simulink model "ame532Project1_GimbalDynamicsModel"  (R2023a)
settings: Solver=ode4  StartTime=0.0  StopTime=10  FixedStep=0.01  RelTol=1e-3
model workspace (MAT data in the model file):
  theta : Simulink.Parameter (value not decoded)
values from neighbouring files (symbols this model uses):
  AR_s2 = b_s2/c_s2    [computeSurfacePos.m]
  AR_s3 = b_s3/c_s3    [computeSurfacePos.m]
  AR_s4 = b_s4/c_s4    [computeSurfacePos.m]
  AR_s5 = b_s5/c_s5    [computeSurfacePos.m]
  area_s2 = c_s2 * b_s2    [computeSurfacePos.m]
  area_s3 = c_s3 * b_s3    [computeSurfacePos.m]
  area_s4 = c_s4 * b_s4    [computeSurfacePos.m]
  area_s5 = c_s5 * b_s5    [computeSurfacePos.m]
  c_s2 = componentMassesAndGeom(3,2)    [computeSurfacePos.m]
  c_s3 = componentMassesAndGeom(4,2)    [computeSurfacePos.m]
  c_s4 = componentMassesAndGeom(1,2)    [computeSurfacePos.m]
  c_s5 = componentMassesAndGeom(2,2)    [computeSurfacePos.m]
undefined symbols (not defined in the file or in its folder): a0_s2, a0_s3, a0_s4, a0_s5, CD0_s2, CD0_s3, CD0_s4, CD0_s5, CDa_s2, CDa_s3, CDa_s4, CDa_s5, CL0_s2, CL0_s3, CL0_s4, CL0_s5, CM0_s2, CM0_s3, CM0_s4, CM0_s5, CMa_s2, CMa_s3, CMa_s4, CMa_s5, e_s2, e_s3, e_s4, e_s5, earthRadius, i_s2, i_s3, i_s4, i_s5, Jxx, Jxy, Jxz, Jyx, Jyy, Jyz, Jzx, Jzy, Jzz, LL, MM, n_s2, n_s3, n_s4, n_s5, NN, rEarth, ro, x_S2_B_B, x_S3_B_B, x_S4_B_B, x_S5_B_B
libraries: simulink_extras x34, matrix_library x22, aerolibutil x7, aerolibfltsims x4, vrlib x3, aerolibtransform2 x2, slpidlib x1, sharedutil x1, simulink x1
(part 3 of 4)

== system ame532Project1_GimbalDynamicsModel/JeoIMUmodel/Aero Forces and Moments/F&M Horiz Stab Surface (S3) ==
  v_B_E_B : Inport
  V_B_A_B (Relative AIr Speed) : Inport  Port=2
  Compute Aero Lift and Drag : MATLAB Function  TreatAsAtomicUnit=on
  Compute Aero Moment : MATLAB Function  TreatAsAtomicUnit=on
  Constant : Constant  Value=[AR_s3 i_s3 CL0_s3 CD0_s3 CDa_s3 a0_s3 e_s3 ro area_s3]
  Constant1 : Constant  Value=[CM0_s3; CMa_s3; c_s3]
  Constant2 : Constant  Value=n_s3
  Demux : Demux  Outputs=9
  Demux1 : Demux  Outputs=3
  F&M in Body : Subsystem
  momS3_B : Outport
  LiftAndDragForceS3_B : Outport  Port=2
  wires:
  Compute Aero Lift and Drag/2(liftSurf) -> F&M in Body/2(Lift)  "Lift Force w.r.t Wind"
  Compute Aero Moment/1(momSurf) -> F&M in Body/1(momSurf)  "Moment of Surface w.r.t Wind"
  Compute Aero Lift and Drag/3(dragSurf) -> F&M in Body/3(Drag)  "Drag Force w.r.t Wind"
  F&M in Body/2(LiftAndDragForceS3_B) -> LiftAndDragForceS3_B/1
  Compute Aero Lift and Drag/1(alphaLocal) -> Compute Aero Moment/2(alphaLocal)
  v_B_E_B/1 -> Compute Aero Lift and Drag/1(v_B_E_B), F&M in Body/4(v_B_E_B), Compute Aero Moment/1(v_B_E_B)
  F&M in Body/1(momS3_B) -> momS3_B/1
  V_B_A_B (Relative AIr Speed)/1 -> Compute Aero Lift and Drag/2(v_B_A_B)
  Constant/1 -> Demux/1
  Demux/1 -> Compute Aero Lift and Drag/3(AR_s3)  "AR_s3"
  Demux/2 -> Compute Aero Lift and Drag/4(i_s3)  "i_s3"
  Constant2/1 -> F&M in Body/5(n_s3), Compute Aero Lift and Drag/5(n_s3)  "n_s3"
  Demux/3 -> Compute Aero Lift and Drag/6(CL0_s3)  "CL0_s3"
  Demux/4 -> Compute Aero Lift and Drag/7(CD0_s3)  "CD0_s3"
  Demux/5 -> Compute Aero Lift and Drag/8(CDa_s3)  "CDa_s3"
  Demux/6 -> Compute Aero Lift and Drag/9(a0_s3)  "a0_s3"
  Demux/7 -> Compute Aero Lift and Drag/10(e_s3)  "e_s3"
  Demux/8 -> Compute Aero Moment/5(ro), Compute Aero Lift and Drag/11(ro)  "ro"
  Demux/9 -> Compute Aero Moment/6(area_s3), Compute Aero Lift and Drag/12(area_s3)  "area_s3"
  Constant1/1 -> Demux1/1
  Demux1/1 -> Compute Aero Moment/3(CM0_s3)  "CMo_s3"
  Demux1/2 -> Compute Aero Moment/4(CMa_s3)  "CMa_s3"
  Demux1/3 -> Compute Aero Moment/7(c_s3)  "c_s3"

== system ame532Project1_GimbalDynamicsModel/JeoIMUmodel/Aero Forces and Moments/F&M Right Wing and Servo Surface (S4) ==
  v_B_E_B : Inport
  V_B_A_B (Relative AIr Speed) : Inport  Port=2
  Compute Aero Lift and Drag : MATLAB Function  TreatAsAtomicUnit=on
  Compute Aero Moment : MATLAB Function  TreatAsAtomicUnit=on
  Constant : Constant  Value="[AR_s4 i_s4  CL0_s4 CD0_s4 CDa_s4 a0_s4 e_s4 ro area_s4]"
  Constant1 : Constant  Value=[CM0_s4; CMa_s4; c_s4]
  Demux : Demux  Outputs=9
  Demux1 : Demux  Outputs=3
  F&M in Body : Subsystem
  n_s4 : Constant  Value=n_s4
  momS4_B : Outport
  LiftAndDragForceS4_B : Outport  Port=2
  wires:
  Compute Aero Lift and Drag/2(liftSurf) -> F&M in Body/2(Lift)  "Lift Force w.r.t Wind"
  Compute Aero Moment/1(momSurf) -> F&M in Body/1(momSurf)  "Moment of Surface w.r.t Wind"
  Compute Aero Lift and Drag/3(dragSurf) -> F&M in Body/3(Drag)  "Drag Force w.r.t Wind"
  F&M in Body/2(LiftAndDragForceS4_B) -> LiftAndDragForceS4_B/1
  Compute Aero Lift and Drag/1(alphaLocal) -> Compute Aero Moment/2(alphaLocal)
  v_B_E_B/1 -> Compute Aero Lift and Drag/1(v_B_E_B), F&M in Body/4(v_B_E_B), Compute Aero Moment/1(v_B_E_B)
  F&M in Body/1(momS4_B) -> momS4_B/1
  V_B_A_B (Relative AIr Speed)/1 -> Compute Aero Lift and Drag/2(v_B_A_B)
  Constant/1 -> Demux/1
  Demux/1 -> Compute Aero Lift and Drag/3(AR_s4)  "AR_s4"
  Demux/2 -> Compute Aero Lift and Drag/4(i_s4)  "i_s4"
  n_s4/1 -> F&M in Body/5(n_s4), Compute Aero Lift and Drag/5(n_s4)  "n_s4"
  Demux/3 -> Compute Aero Lift and Drag/6(CL0_s4)  "CL0_s4"
  Demux/4 -> Compute Aero Lift and Drag/7(CD0_s4)  "CD0_s4"
  Demux/5 -> Compute Aero Lift and Drag/8(CDa_s4)  "CDa_s4"
  Demux/6 -> Compute Aero Lift and Drag/9(a0_s4)  "a0_s4"
  Demux/7 -> Compute Aero Lift and Drag/10(e_s4)  "e_s4"
  Demux/9 -> Compute Aero Moment/6(area_s4), Compute Aero Lift and Drag/12(area_s4)  "area_s4"
  Constant1/1 -> Demux1/1
  Demux1/1 -> Compute Aero Moment/3(CM0_s4)  "CMo_s4"
  Demux1/2 -> Compute Aero Moment/4(CMa_s4)  "CMa_s4"
  Demux1/3 -> Compute Aero Moment/7(c_s4)  "c_s4"
  Demux/8 -> Compute Aero Moment/5(ro), Compute Aero Lift and Drag/11(ro)  "e_s4"

== system ame532Project1_GimbalDynamicsModel/JeoIMUmodel/Aero Forces and Moments/F&M Right Wing and Servo Surface (S5) ==
  v_B_E_B : Inport
  V_B_A_B (Relative AIr Speed) : Inport  Port=2
  Compute Aero Lift and Drag : MATLAB Function  TreatAsAtomicUnit=on
  Compute Aero Moment : MATLAB Function  TreatAsAtomicUnit=on
  Constant : Constant  Value=[AR_s5 i_s5 CL0_s5 CD0_s5 CDa_s5 a0_s5 e_s5 ro area_s5]
  Constant1 : Constant  Value=[CM0_s5; CMa_s5; c_s5]
  Demux : Demux  Outputs=9
  Demux1 : Demux  Outputs=3
  F&M in Body : Subsystem
  n_s5 : Constant  Value=n_s5
  momS5_B : Outport
  LiftAndDragForceS5_B : Outport  Port=2
  wires:
  Compute Aero Lift and Drag/2(liftSurf) -> F&M in Body/2(Lift)  "Lift Force w.r.t Wind"
  Compute Aero Moment/1(momSurf) -> F&M in Body/1(momSurf)  "Moment of Surface w.r.t Wind"
  Compute Aero Lift and Drag/3(dragSurf) -> F&M in Body/3(Drag)  "Drag Force w.r.t Wind"
  F&M in Body/2(LiftAndDragForceS5_B) -> LiftAndDragForceS5_B/1
  Compute Aero Lift and Drag/1(alphaLocal) -> Compute Aero Moment/2(alphaLocal)
  v_B_E_B/1 -> Compute Aero Lift and Drag/1(v_B_E_B), F&M in Body/4(v_B_E_B), Compute Aero Moment/1(v_B_E_B)
  F&M in Body/1(momS5_B) -> momS5_B/1
  V_B_A_B (Relative AIr Speed)/1 -> Compute Aero Lift and Drag/2(v_B_A_B)
  Constant/1 -> Demux/1
  Demux/1 -> Compute Aero Lift and Drag/3(AR_s5)  "AR_s5"
  Demux/2 -> Compute Aero Lift and Drag/4(i_s5)  "i_s5"
  n_s5/1 -> F&M in Body/5(n_s5), Compute Aero Lift and Drag/5(n_s5)  "n_s5"
  Demux/3 -> Compute Aero Lift and Drag/6(CL0_s5)  "CL0_s5"
  Demux/4 -> Compute Aero Lift and Drag/7(CD0_s5)  "CD0_s5"
  Demux/5 -> Compute Aero Lift and Drag/8(CDa_s5)  "CDa_s5"
  Demux/6 -> Compute Aero Lift and Drag/9(a0_s5)  "a0_s5"
  Demux/7 -> Compute Aero Lift and Drag/10(e_s5)  "e_s5"
  Demux/8 -> Compute Aero Moment/5(ro), Compute Aero Lift and Drag/11(ro)  "ro"
  Demux/9 -> Compute Aero Moment/6(area_s5), Compute Aero Lift and Drag/12(area_s5)  "area_s5"
  Constant1/1 -> Demux1/1
  Demux1/1 -> Compute Aero Moment/3(CM0_s5)  "CMo_s5"
  Demux1/2 -> Compute Aero Moment/4(CMa_s5)  "CMa_s5"
  Demux1/3 -> Compute Aero Moment/7(c_s5)  "c_s5"

== system ame532Project1_GimbalDynamicsModel/JeoIMUmodel/Rotational Dynamics/Using Cross Product Matrix ==
  wPQR : Inport
  J Matrix : Inport  Port=2
  Matrix Multiply : Product  Multiplication=Matrix(*)
  Matrix Multiply1 : Product  Multiplication=Matrix(*)
  Omega Cross Matrix : MATLAB Function  TreatAsAtomicUnit=on
  OmegaJw : Outport
  wires:
  wPQR/1 -> Omega Cross Matrix/1(PQR), Matrix Multiply1/2
  J Matrix/1 -> Matrix Multiply1/1
  Omega Cross Matrix/1(omegaMat) -> Matrix Multiply/1
  Matrix Multiply1/1 -> Matrix Multiply/2  "Jw"
  Matrix Multiply/1 -> OmegaJw/1

== system ame532Project1_GimbalDynamicsModel/JeoIMUmodel/Rotational Dynamics/Using Cross Product Operator Only ==
  wPQR : Inport
  J Matrix : Inport  Port=2
  Cross Product : matrix_library/Cross Product
  Matrix Multiply1 : Product  Multiplication=Matrix(*)
  OmegaJw : Outport
  wires:
  wPQR/1 -> Matrix Multiply1/2, Cross Product/1
  J Matrix/1 -> Matrix Multiply1/1
  Matrix Multiply1/1 -> Cross Product/2  "Jw"
  Cross Product/1 -> OmegaJw/1

== system ame532Project1_GimbalDynamicsModel/JeoIMUmodel/TransKin_RotKin_TansDynam/Rotational Kinematics_Euler ==
  wVectorBodyRates_PQR : Inport
  Demux : Demux  Outputs=3
  HinvMatrix : MATLAB Function  TreatAsAtomicUnit=on
  Initial Attitude_rad w.r.t ECEF : Constant  Value=[0; 0; 0]
  Integrator : Integrator  InitialConditionSource=external  InitialCondition=[0;30;30]
  MatrixMultiply : Product  Multiplication=Matrix(*)
  Scope : Scope
  Terminator : Terminator
  Theta Vector_rad : Outport
  wires:
  HinvMatrix/1(hinv) -> MatrixMultiply/1
  MatrixMultiply/1 -> Integrator/1  "Theta Vector Dot"
  Integrator/1 -> Demux/1, Theta Vector_rad/1, Scope/1  "Theta Vector_rad"
  Demux/1 -> HinvMatrix/2(rollPhi)  "roll_rad"
  Demux/2 -> HinvMatrix/1(pitchTheta)  "pitch_rad"
  Demux/3 -> Terminator/1  "yaw_rad"
  wVectorBodyRates_PQR/1 -> MatrixMultiply/2  "wVector Body Rates_PQR"
  Initial Attitude_rad w.r.t ECEF/1 -> Integrator/2

== system ame532Project1_GimbalDynamicsModel/JeoIMUmodel/TransKin_RotKin_TansDynam/Translational Dynamics ==
  C_B_N : Inport
  wBodyRates_PQR : Inport  Port=2
  Aero Forces : Inport  Port=3
  Accelerometer : Subsystem
  Cross Product : matrix_library/Cross Product
  E_xdot_B_E_B_xComp_mPs : Constant  Commented=on  Value=150
  E_xdot_B_E_B_yComp_mPs : Constant  Commented=on  Value=0
  E_xdot_B_E_B_zComp_mPs : Constant  Commented=on  Value=0
  External Forces_mPsec^2_xComp_wrtB : Constant  Value=0
  External Forces_mPsec^2_yComp_wrtB : Constant  Value=0
  External Forces_mPsec^2_zComp_wrtB : Constant  Value=0
  Gain : Gain  Gain=-1
  Initial Body Velocity : Constant  Value=[13; 0; 0]
  Integrator : Integrator  InitialConditionSource=external  InitialCondition=[50;0;0]
  Manual Switch : ManualSwitch
  Manual Switch1 : ManualSwitch  CurrentSetting=0
  Matrix Multiply : Product  Multiplication=Matrix(*)
  Sum : Sum  Inputs=|+++
  Terminator : Terminator  Commented=on
  Vector Concatenate : Concatenate  Commented=on  NumInputs=3  Mode=Multidimensional array
  Vector Concatenate1 : Concatenate  NumInputs=3
  Vector Concatenate2 : Concatenate  NumInputs=3
  gravity_mPsec^2_xComp_wrtN : Constant  Value=0
  gravity_mPsec^2_yComp_wrtN : Constant  Value=0
  gravity_mPsec^2_zComp_wrtN : Constant  Value=9.8
  E_xdot_B_E_B : Outport
  wires:
  E_xdot_B_E_B_xComp_mPs/1 -> Vector Concatenate/1
  E_xdot_B_E_B_zComp_mPs/1 -> Vector Concatenate/3
  E_xdot_B_E_B_yComp_mPs/1 -> Vector Concatenate/2
  Vector Concatenate/1 -> Terminator/1  "E_xdot_B_E_B"
  External Forces_mPsec^2_xComp_wrtB/1 -> Vector Concatenate2/1
  gravity_mPsec^2_xComp_wrtN/1 -> Vector Concatenate1/1
  wBodyRates_PQR/1 -> Cross Product/1
  Cross Product/1 -> Gain/1  "Vdot_B_E_B"
  Integrator/1 -> E_xdot_B_E_B/1, Cross Product/2  "V_B_E_B"
  Gain/1 -> Sum/3
  Sum/1 -> Manual Switch1/2, Accelerometer/1(True Acceleration)  "True Vdot_B_E_B"
  gravity_mPsec^2_yComp_wrtN/1 -> Vector Concatenate1/2
  gravity_mPsec^2_zComp_wrtN/1 -> Vector Concatenate1/3
  Vector Concatenate1/1 -> Matrix Multiply/2
  External Forces_mPsec^2_yComp_wrtB/1 -> Vector Concatenate2/2
  External Forces_mPsec^2_zComp_wrtB/1 -> Vector Concatenate2/3
  Vector Concatenate2/1 -> Manual Switch/2
  C_B_N/1 -> Matrix Multiply/1  "c_B_N"
  Matrix Multiply/1 -> Sum/2
  Aero Forces/1 -> Manual Switch/1
  Manual Switch/1 -> Sum/1
  Initial Body Velocity/1 -> Integrator/2
  Accelerometer/1(Measured Acceleration) -> Manual Switch1/1  "measured Vdot_B_E_B"
  Manual Switch1/1 -> Integrator/1

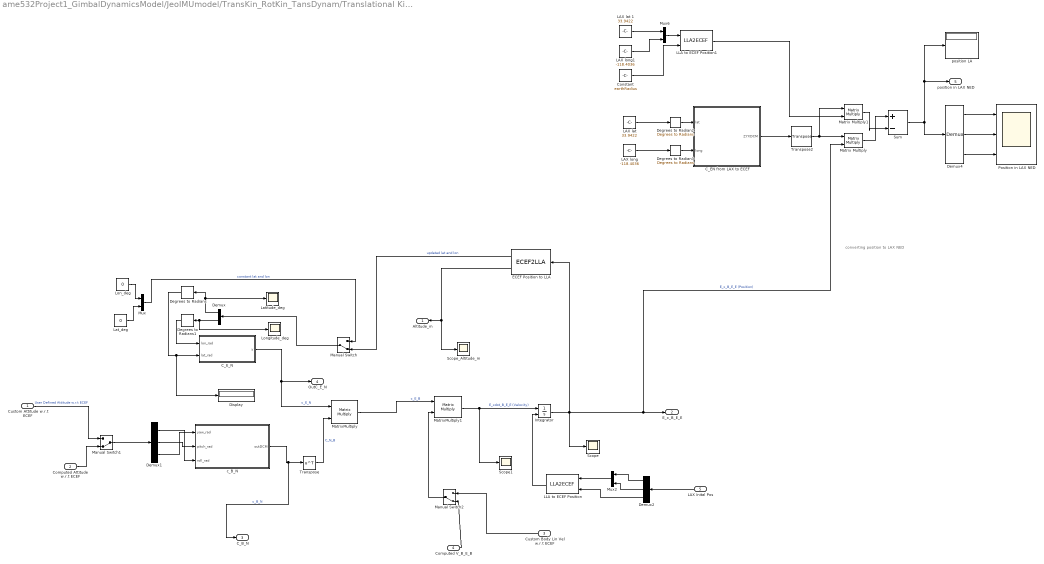
== system ame532Project1_GimbalDynamicsModel/JeoIMUmodel/TransKin_RotKin_TansDynam/Translational Kinematics ==
  note: converting position to LAX NED
  Custom Attitude w.r.t ECEF : Inport
  Computed Attitude w.r.t ECEF : Inport  Port=2
  Custom Body Lin Vel w.r.t ECEF : Inport  Port=3
  Computed V_B_E_B : Inport  Port=4
  LAX Inital Pos : Inport  Port=5
  C_EN from LAX to ECEF : MATLAB Function  TreatAsAtomicUnit=on
  C_E_N : MATLAB Function  TreatAsAtomicUnit=on
  Constant : Constant  Value=earthRadius
  Degrees to Radian2 : simulink_extras/Transformations/Degrees to Radians
  Degrees to Radian3 : simulink_extras/Transformations/Degrees to Radians
  Degrees to Radians : simulink_extras/Transformations/Degrees to Radians
  Degrees to Radians1 : simulink_extras/Transformations/Degrees to Radians
  Demux : Demux  Outputs=2
  Demux1 : Demux  Outputs=3
  Demux2 : Demux  Outputs=3
  Demux4 : Demux  Outputs=3
  Display : Display
  ECEF Position to LLA : ECEF2LLA  ptype=Custom
  Integrator : Integrator  InitialConditionSource=external  InitialCondition=[0;0;rEarth]
  "LAX lat " : Constant  Value=33.9422
  LAX lat 1 : Constant  Value=33.9422
  LAX long : Constant  Value=-118.4036
  LAX long1 : Constant  Value=-118.4036
  LLA to ECEF Position : LLA2ECEF  ptype=Custom
  LLA to ECEF Position1 : LLA2ECEF
  Lat_deg : Constant  Value=0
  Latitude_deg : Scope
  Lon_deg : Constant  Value=0
  Longitude_deg : Scope
  Manual Switch : ManualSwitch  CurrentSetting=0
  Manual Switch1 : ManualSwitch  CurrentSetting=0
  Manual Switch2 : ManualSwitch  CurrentSetting=0
  Matrix Multiply : Product  Multiplication=Matrix(*)
  Matrix Multiply1 : Product  Multiplication=Matrix(*)
  MatrixMultiply : Product  Multiplication=Matrix(*)
  MatrixMultiply1 : Product  Multiplication=Matrix(*)
  Mux : Mux  Inputs=2
  Mux2 : Mux  Inputs=2
  Mux6 : Mux  Inputs=2
  Position in LAX NED : Scope  NumInputPorts=3
  Scope : Scope
  Scope1 : Scope
  Scope_Altitude_m : Scope
  Sum : Sum  Inputs=|+-
  Transpose : Math  Operator=transpose
  Transpose2 : matrix_library/Transpose
  c_B_N : MATLAB Function  TreatAsAtomicUnit=on
  "position LA " : Display
  Altitude_m : Outport
  E_x_B_E_E : Outport  Port=2
  C_B_N : Outport  Port=3
  OutC_E_N : Outport  Port=4
  position in LAX NED : Outport  Port=5
  wires:
  MatrixMultiply1/1 -> Scope1/1, Integrator/1  "E_xdot_B_E_E (Velocity)"
  C_E_N/1(y) -> OutC_E_N/1, MatrixMultiply/1  "c_E_N"
  Manual Switch1/1 -> Demux1/1
  MatrixMultiply/1 -> MatrixMultiply1/1  "c_E_B"
  Degrees to Radians/1 -> Display/1, C_E_N/2(lat_rad)
  ECEF Position to LLA/2 -> Altitude_m/1, Scope_Altitude_m/1
  Transpose/1 -> MatrixMultiply/2  "C_N_B"
  Lon_deg/1 -> Mux/1
  Mux/1 -> Manual Switch/1  "constant lat and lon"
  Lat_deg/1 -> Mux/2
  Integrator/1 -> ECEF Position to LLA/1, Matrix Multiply/2, E_x_B_E_E/1, Scope/1  "E_x_B_E_E (Position)"
  ECEF Position to LLA/1 -> Manual Switch/2  "updated lat and lon"
  Demux1/3 -> c_B_N/1(yaw_rad)
  Demux1/1 -> c_B_N/3(roll_rad)
  Demux1/2 -> c_B_N/2(pitch_rad)
  c_B_N/1(outDCM) -> C_B_N/1, Transpose/1  "c_B_N"
  Manual Switch/1 -> Demux/1
  Manual Switch2/1 -> MatrixMultiply1/2
  Custom Attitude w.r.t ECEF/1 -> Manual Switch1/1  "User Defined Attitude w.r.t ECEF"
  Computed Attitude w.r.t ECEF/1 -> Manual Switch1/2
  Custom Body Lin Vel w.r.t ECEF/1 -> Manual Switch2/1
  Computed V_B_E_B/1 -> Manual Switch2/2
  Demux/2 -> Longitude_deg/1, Degrees to Radians1/1
  Demux/1 -> Degrees to Radians/1, Latitude_deg/1
  Degrees to Radians1/1 -> C_E_N/1(lon_rad)
  LAX Inital Pos/1 -> Demux2/1
  Demux2/1 -> Mux2/1
  Demux2/2 -> Mux2/2
  Demux2/3 -> LLA to ECEF Position/2
  Mux2/1 -> LLA to ECEF Position/1
  LLA to ECEF Position/1 -> Integrator/2
  LLA to ECEF Position1/1 -> Matrix Multiply1/2
  LAX long1/1 -> Mux6/2
  Matrix Multiply/1 -> Sum/1
  Demux4/2 -> Position in LAX NED/2
  Mux6/1 -> LLA to ECEF Position1/1
  Matrix Multiply1/1 -> Sum/2
  Constant/1 -> LLA to ECEF Position1/2
  LAX lat 1/1 -> Mux6/1
  Demux4/3 -> Position in LAX NED/3
  Demux4/1 -> Position in LAX NED/1
  C_EN from LAX to ECEF/1(ZYXDCM) -> Transpose2/1
  "LAX lat "/1 -> Degrees to Radian2/1
  Transpose2/1 -> Matrix Multiply1/1, Matrix Multiply/1
  LAX long/1 -> Degrees to Radian3/1
  Degrees to Radian2/1 -> C_EN from LAX to ECEF/1(lat)
  Degrees to Radian3/1 -> C_EN from LAX to ECEF/2(long)
  Sum/1 -> "position LA "/1, position in LAX NED/1, Demux4/1

== system ame532Project1_GimbalDynamicsModel/JeoIMUmodel/Aero Forces and Moments/F&M Horiz Stab Surface (S2)/F&M in Body ==
  momSurf : Inport
  Lift : Inport  Port=2
  Drag : Inport  Port=3
  v_B_E_B : Inport  Port=4
  n_s2 : Inport  Port=5
  Constant : Constant  Value=x_S2_B_B
  Force Due to Lift and Drag : MATLAB Function  TreatAsAtomicUnit=on
  Moment S2 : MATLAB Function  TreatAsAtomicUnit=on
  momS2_B : Outport
  LiftAndDragForceS2_B : Outport  Port=2
  wires:
  momSurf/1 -> Moment S2/1(momSurf)
  Lift/1 -> Force Due to Lift and Drag/1(lift)
  Drag/1 -> Force Due to Lift and Drag/2(drag)
  Force Due to Lift and Drag/1(forceLiftDragS2_B) -> Moment S2/2(FliftdragS), LiftAndDragForceS2_B/1
  v_B_E_B/1 -> Force Due to Lift and Drag/3(v_B_E_B)
  Moment S2/1(momS2_B) -> momS2_B/1
  n_s2/1 -> Force Due to Lift and Drag/4(n_s2), Moment S2/3(n_s2)
  Constant/1 -> Moment S2/4(x_S2_B_B)

== system ame532Project1_GimbalDynamicsModel/JeoIMUmodel/Aero Forces and Moments/F&M Horiz Stab Surface (S3)/F&M in Body ==
  momSurf : Inport
  Lift : Inport  Port=2
  Drag : Inport  Port=3
  v_B_E_B : Inport  Port=4
  n_s3 : Inport  Port=5
  Constant : Constant  Value=x_S3_B_B
  Force Due to Lift and Drag : MATLAB Function  TreatAsAtomicUnit=on
  Moment S3 : MATLAB Function  TreatAsAtomicUnit=on
  momS3_B : Outport
  LiftAndDragForceS3_B : Outport  Port=2
  wires:
  momSurf/1 -> Moment S3/1(momSurf)
  Lift/1 -> Force Due to Lift and Drag/1(lift)
  Drag/1 -> Force Due to Lift and Drag/2(drag)
  Force Due to Lift and Drag/1(forceLiftDragS3_B) -> Moment S3/2(FliftdragS), LiftAndDragForceS3_B/1
  v_B_E_B/1 -> Force Due to Lift and Drag/3(v_B_E_B)
  Moment S3/1(momS3_B) -> momS3_B/1
  n_s3/1 -> Force Due to Lift and Drag/4(n_s3), Moment S3/3(n_s3)
  Constant/1 -> Moment S3/4(x_S3_B_B)

== system ame532Project1_GimbalDynamicsModel/JeoIMUmodel/Aero Forces and Moments/F&M Right Wing and Servo Surface (S4)/F&M in Body ==
  momSurf : Inport
  Lift : Inport  Port=2
  Drag : Inport  Port=3
  v_B_E_B : Inport  Port=4
  n_s4 : Inport  Port=5
  Constant : Constant  Value=x_S4_B_B
  Force Due to Lift and Drag : MATLAB Function  TreatAsAtomicUnit=on
  Moment S4 : MATLAB Function  TreatAsAtomicUnit=on
  momS4_B : Outport
  LiftAndDragForceS4_B : Outport  Port=2
  wires:
  momSurf/1 -> Moment S4/1(momSurf)
  Lift/1 -> Force Due to Lift and Drag/1(lift)
  Drag/1 -> Force Due to Lift and Drag/2(drag)
  Force Due to Lift and Drag/1(forceLiftDragS4_B) -> Moment S4/2(FliftdragS), LiftAndDragForceS4_B/1
  v_B_E_B/1 -> Force Due to Lift and Drag/3(v_B_E_B)
  Moment S4/1(momS4_B) -> momS4_B/1
  n_s4/1 -> Force Due to Lift and Drag/4(n_s4), Moment S4/3(n_s4)
  Constant/1 -> Moment S4/4(x_S4_B_B)

== system ame532Project1_GimbalDynamicsModel/JeoIMUmodel/Aero Forces and Moments/F&M Right Wing and Servo Surface (S5)/F&M in Body ==
  momSurf : Inport
  Lift : Inport  Port=2
  Drag : Inport  Port=3
  v_B_E_B : Inport  Port=4
  n_s5 : Inport  Port=5
  Constant : Constant  Value=x_S5_B_B
  Force Due to Lift and Drag : MATLAB Function  TreatAsAtomicUnit=on
  Moment S5 : MATLAB Function  TreatAsAtomicUnit=on
  momS5_B : Outport
  LiftAndDragForceS5_B : Outport  Port=2
  wires:
  momSurf/1 -> Moment S5/1(momSurf)
  Lift/1 -> Force Due to Lift and Drag/1(lift)
  Drag/1 -> Force Due to Lift and Drag/2(drag)
  Force Due to Lift and Drag/1(forceLiftDragS5_B) -> Moment S5/2(FliftdragS), LiftAndDragForceS5_B/1
  v_B_E_B/1 -> Force Due to Lift and Drag/3(v_B_E_B)
  Moment S5/1(momS5_B) -> momS5_B/1
  n_s5/1 -> Force Due to Lift and Drag/4(n_s5), Moment S5/3(n_s5)
  Constant/1 -> Moment S5/4(x_S5_B_B)

== system ame532Project1_GimbalDynamicsModel/JeoIMUmodel/TransKin_RotKin_TansDynam/Translational Dynamics/Accelerometer ==
  True Acceleration : Inport
  Band-Limited White Noise : simulink/Sources/Band-Limited White Noise  Cov=[0.000001]  Ts=0.1  seed=[23341]
  Bias : Constant  Value=[0.025*9.8 0.025*9.8 0.025*9.8]
  Scale Factor : Gain  Gain=0.001
  Sum : Sum  Inputs=|++
  Sum1 : Sum  Inputs=|++
  Measured Acceleration : Outport
  wires:
  True Acceleration/1 -> Sum/1
  Bias/1 -> Sum/2
  Sum/1 -> Scale Factor/1
  Scale Factor/1 -> Sum1/1
  Band-Limited White Noise/1 -> Sum1/2
  Sum1/1 -> Measured Acceleration/1

== matlab function ame532Project1_GimbalDynamicsModel/Gimbal Aircraft dynamic sim/Rotational Kinematics/C_EN2 ==
  data: roll input; ZYXDCM output; pitch input; yaw input
function ZYXDCM = DCM_from_Euler(roll,pitch,yaw) % sequence is yaw pitch roll
    yaw_matrix = [cos(yaw) -sin(yaw) 0;
                  sin(yaw) cos(yaw) 0;
                  0 0 1];
    pitch_matrix = [cos(pitch) 0 sin(pitch);
                    0           1           0;
                    -sin(pitch) 0  cos(pitch)];
    roll_matrix = [1            0           0;
                    0          cos(roll)    -sin(roll);
                    0           sin(roll)  cos(roll)];
    ZYXDCM = roll_matrix*pitch_matrix*yaw_matrix;
end

== matlab function ame532Project1_GimbalDynamicsModel/Gimbal system/Rotational Kinematics/MATLAB Function2 ==
  data: phi input; H_matrix_inv output; theta input; psi input
function H_matrix_inv = inv_h_matrix_from_euler(phi,theta,psi)

H_matrix_inv = [1, tan(theta)*sin(phi), tan(theta)*cos(phi);
                0,      cos(phi),           -sin(phi);      
                0,     sin(phi)/cos(theta),   cos(phi)/cos(theta)];

end

== matlab function ame532Project1_GimbalDynamicsModel/Gimbal system/Rotational Kinematics/MATLAB Function3 ==
  data: p input; Cross_Product_Matrix output; q input; r input
function Cross_Product_Matrix = omega_to_cross_product_matrix(p,q,r)

    Cross_Product_Matrix =[0 -r q; r 0 -p; -q p 0];

end

== matlab function ame532Project1_GimbalDynamicsModel/Gimbal system/Rotational Kinematics/MATLAB Function4 ==
  data: DCM input; roll output; pitch output; yaw output
function [roll, pitch, yaw] = Euler_from_DCM(DCM)
   roll = atan2(DCM(2,3),DCM(3,3));
   pitch = -asin(DCM(1,3));
   yaw = atan2(DCM(1,2),DCM(1,1));
end

== matlab function ame532Project1_GimbalDynamicsModel/Gimbal system/Rotational Kinematics/MATLAB Function5 ==
  data: DCM input; roll output; pitch output; yaw output
function [roll, pitch, yaw] = Euler_from_DCM(DCM)
   roll = atan2(DCM(2,3),DCM(3,3));
   pitch = asin(DCM(1,3));
   yaw = atan2(DCM(1,2),DCM(1,1));
end

== matlab function ame532Project1_GimbalDynamicsModel/Gimbal system/Rotational Kinematics/MATLAB Function6 ==
  data: DCM input; roll output; pitch output; yaw output
function [roll, pitch, yaw] = Euler_from_DCM(DCM)
   roll = atan2(DCM(2,3),DCM(3,3));
   pitch = -asin(DCM(1,3));
   yaw = atan2(DCM(1,2),DCM(1,1));
end

== matlab function ame532Project1_GimbalDynamicsModel/Gimbal system/Rotational Kinematics/MATLAB Function7 ==
  data: quat input; roll output; pitch output; yaw output
function [roll, pitch, yaw] = Euler_from_Quat(quat)
    DCM = zeros(3,3);
    DCM(1) = (quat(1)^2+quat(2)^2-quat(3)^2-quat(4)^2);
    DCM(2) = 2*(quat(2)*quat(3)-quat(1)*quat(4));
    DCM(3) = 2*(quat(2)*quat(4)+quat(1)*quat(3));
    DCM(4) = 2*(quat(2)*quat(3)+quat(1)*quat(4));
    DCM(5) = (quat(1)^2-quat(2)^2+quat(3)^2-quat(4)^2);
    DCM(6) = 2*(quat(3)*quat(4)-quat(1)*quat(2));
    DCM(7) = 2*(quat(2)*quat(4)-quat(1)*quat(3));
    DCM(8) = 2*(quat(3)*quat(4)+quat(1)*quat(2));
    DCM(9) = (quat(1)^2-quat(2)^2-quat(3)^2+quat(4)^2);

    roll = atan2(DCM(2,3),DCM(3,3));
    pitch = -asin(DCM(1,3));
    yaw = atan2(DCM(1,2),DCM(1,1));
end

== matlab function ame532Project1_GimbalDynamicsModel/Gimbal system/Rotational Kinematics/MATLAB Function8 ==
  data: roll input; ZYXquat_inv output; pitch input; yaw input; ZYXquat output
function [ZYXquat_inv,ZYXquat] = Quat_from_Euler(roll,pitch,yaw)
    q_yaw = zeros(4,1);
    q_yaw(1) = cos(yaw/2);
    q_yaw(2:4,1) = sin(yaw/2)*[0 0 1]';

    q_pitch = zeros(4,1);
    q_pitch(1) = cos(pitch/2);
    q_pitch(2:4,1) = sin(pitch/2)*[0 1 0]';

    q_roll = zeros(4,1);
    q_roll(1) = cos(roll/2);
    q_roll(2:4,1) = sin(roll/2)*[1 0 0]';
    
    inv_q_yaw = [q_yaw(1);-q_yaw(2:4)];
    inv_q_pitch = [q_pitch(1);-q_pitch(2:4)];
    inv_q_roll = [q_roll(1);-q_roll(2:4)];

    ZYXquat_inv = quat_mult(quat_mult(inv_q_roll,inv_q_pitch),inv_q_yaw);
    ZYXquat = quat_mult(quat_mult(q_yaw,q_pitch),q_roll);

end

function quat = quat_mult(q1,q2)
    quat = zeros(4,1);
    quat(1) = q1(1)*q2(1)-q1(2)*q2(2)-q1(3)*q2(3)-q1(4)*q2(4);
    quat(2) = q1(1)*q2(2)+q1(2)*q2(1)+q1(3)*q2(4)-q1(4)*q2(3);
    quat(3) = q1(1)*q2(3)-q1(2)*q2(4)+q1(3)*q2(1)+q1(4)*q2(2);
    quat(4) = q1(1)*q2(4)+q1(2)*q2(3)-q1(3)*q2(2)+q1(4)*q2(1);
end

== matlab function ame532Project1_GimbalDynamicsModel/Gimbal system/Rotational Kinematics/MATLAB Function9 ==
  data: q1 input; quat output; q2 input
function quat = quat_mult(q1,q2)
    quat = zeros(4,1);
    quat(1) = q1(1)*q2(1)-q1(2)*q2(2)-q1(3)*q2(3)-q1(4)*q2(4);
    quat(2) = q1(1)*q2(2)+q1(2)*q2(1)+q1(3)*q2(4)-q1(4)*q2(3);
    quat(3) = q1(1)*q2(3)-q1(2)*q2(4)+q1(3)*q2(1)+q1(4)*q2(2);
    quat(4) = q1(1)*q2(4)+q1(2)*q2(3)-q1(3)*q2(2)+q1(4)*q2(1);
end

== matlab function ame532Project1_GimbalDynamicsModel/Gimbal system/Rotational Kinematics/MATLAB Function ==
  data: theta input; H output
function H = HpitchDCM(theta)

H = [cos(theta) 0 -sin(theta); 0 1 0; sin(theta) 0 cos(theta)];

%H = [0 0 0; 0 1 0; sin(theta) 0 cos(theta)];

end

== matlab function ame532Project1_GimbalDynamicsModel/Gimbal system/DCM_C_OG ==
  data: roll input; ZYXDCM output; pitch input; yaw input
function ZYXDCM = DCM_from_Euler(roll,pitch,yaw) % sequence is yaw pitch roll
    yaw_matrix = [cos(-yaw) sin(-yaw) 0;
                  -sin(-yaw) cos(-yaw) 0;
                  0 0 1];
    pitch_matrix = [cos(-pitch) 0 -sin(-pitch);
                    0           1           0;
                    sin(-pitch) 0  cos(-pitch)];
    roll_matrix = [1            0           0;
                    0          cos(roll)    sin(roll);
                    0           -sin(roll)  cos(roll)];
    ZYXDCM = pitch_matrix*yaw_matrix;
end

== matlab function ame532Project1_GimbalDynamicsModel/Gimbal Aircraft dynamic sim/Rotational Kinematics/MATLAB Function5 ==
  data: DCM input; roll output; pitch output; yaw output
function [roll, pitch, yaw] = Euler_from_DCM(DCM)
   roll = atan2(DCM(2,3),DCM(3,3));
   pitch = asin(DCM(1,3));
   yaw = atan2(DCM(1,2),DCM(1,1));
end

== matlab function ame532Project1_GimbalDynamicsModel/Gimbal Aircraft dynamic sim/Rotational Kinematics/MATLAB Function6 ==
  data: DCM input; roll output; pitch output; yaw output
function [roll, pitch, yaw] = Euler_from_DCM(DCM)
   roll = atan2(DCM(2,3),DCM(3,3));
   pitch = -asin(DCM(1,3));
   yaw = atan2(DCM(1,2),DCM(1,1));
end

== matlab function ame532Project1_GimbalDynamicsModel/Gimbal Aircraft dynamic sim/Rotational Kinematics/MATLAB Function7 ==
  data: quat input; roll output; pitch output; yaw output
function [roll, pitch, yaw] = Euler_from_Quat(quat)
    DCM = zeros(3,3);
    DCM(1) = (quat(1)^2+quat(2)^2-quat(3)^2-quat(4)^2);
    DCM(2) = 2*(quat(2)*quat(3)-quat(1)*quat(4));
    DCM(3) = 2*(quat(2)*quat(4)+quat(1)*quat(3));
    DCM(4) = 2*(quat(2)*quat(3)+quat(1)*quat(4));
    DCM(5) = (quat(1)^2-quat(2)^2+quat(3)^2-quat(4)^2);
    DCM(6) = 2*(quat(3)*quat(4)-quat(1)*quat(2));
    DCM(7) = 2*(quat(2)*quat(4)-quat(1)*quat(3));
    DCM(8) = 2*(quat(3)*quat(4)+quat(1)*quat(2));
    DCM(9) = (quat(1)^2-quat(2)^2-quat(3)^2+quat(4)^2);

    roll = atan2(DCM(2,3),DCM(3,3));
    pitch = -asin(DCM(1,3));
    yaw = atan2(DCM(1,2),DCM(1,1));
end

== matlab function ame532Project1_GimbalDynamicsModel/Gimbal Aircraft dynamic sim/Rotational Kinematics/C_BN ==
  data: roll input; ZYXDCM output; pitch input; yaw input
function ZYXDCM = DCM_from_Euler(roll,pitch,yaw) % sequence is yaw pitch roll
    yaw_matrix = [cos(yaw) sin(yaw) 0;
                  -sin(yaw) cos(yaw) 0;
                  0 0 1];
    pitch_matrix = [cos(pitch) 0 -sin(pitch);
                    0           1           0;
                    sin(pitch) 0  cos(pitch)];
    roll_matrix = [1            0           0;
                    0          cos(roll)    sin(roll);
                    0           -sin(roll)  cos(roll)];
    ZYXDCM = roll_matrix*pitch_matrix*yaw_matrix;
end

== matlab function ame532Project1_GimbalDynamicsModel/Gimbal Aircraft dynamic sim/Rotational Kinematics/MATLAB Function8 ==
  data: roll input; ZYXquat_inv output; pitch input; yaw input; ZYXquat output
function [ZYXquat_inv,ZYXquat] = Quat_from_Euler(roll,pitch,yaw)
    q_yaw = zeros(4,1);
    q_yaw(1) = cos(yaw/2);
    q_yaw(2:4,1) = sin(yaw/2)*[0 0 1]';

    q_pitch = zeros(4,1);
    q_pitch(1) = cos(pitch/2);
    q_pitch(2:4,1) = sin(pitch/2)*[0 1 0]';

    q_roll = zeros(4,1);
    q_roll(1) = cos(roll/2);
    q_roll(2:4,1) = sin(roll/2)*[1 0 0]';
    
    inv_q_yaw = [q_yaw(1);-q_yaw(2:4)];
    inv_q_pitch = [q_pitch(1);-q_pitch(2:4)];
    inv_q_roll = [q_roll(1);-q_roll(2:4)];

    ZYXquat_inv = quat_mult(quat_mult(inv_q_roll,inv_q_pitch),inv_q_yaw);
    ZYXquat = quat_mult(quat_mult(q_yaw,q_pitch),q_roll);

end

function quat = quat_mult(q1,q2)
    quat = zeros(4,1);
    quat(1) = q1(1)*q2(1)-q1(2)*q2(2)-q1(3)*q2(3)-q1(4)*q2(4);
    quat(2) = q1(1)*q2(2)+q1(2)*q2(1)+q1(3)*q2(4)-q1(4)*q2(3);
    quat(3) = q1(1)*q2(3)-q1(2)*q2(4)+q1(3)*q2(1)+q1(4)*q2(2);
    quat(4) = q1(1)*q2(4)+q1(2)*q2(3)-q1(3)*q2(2)+q1(4)*q2(1);
end

== matlab function ame532Project1_GimbalDynamicsModel/Gimbal Aircraft dynamic sim/Rotational Kinematics/MATLAB Function9 ==
  data: q1 input; quat output; q2 input
function quat = quat_mult(q1,q2)
    quat = zeros(4,1);
    quat(1) = q1(1)*q2(1)-q1(2)*q2(2)-q1(3)*q2(3)-q1(4)*q2(4);
    quat(2) = q1(1)*q2(2)+q1(2)*q2(1)+q1(3)*q2(4)-q1(4)*q2(3);
    quat(3) = q1(1)*q2(3)-q1(2)*q2(4)+q1(3)*q2(1)+q1(4)*q2(2);
    quat(4) = q1(1)*q2(4)+q1(2)*q2(3)-q1(3)*q2(2)+q1(4)*q2(1);
end

== matlab function ame532Project1_GimbalDynamicsModel/Gimbal Aircraft dynamic sim/Unused tranlational kinmatics/C_EN4 ==
  data: roll input; ZYXDCM output; pitch input; yaw input
function ZYXDCM = DCM_from_Euler(roll,pitch,yaw) % sequence is yaw pitch roll
    yaw_matrix = [cos(yaw) sin(yaw) 0;
                  -sin(yaw) cos(yaw) 0;
                  0 0 1];
    pitch_matrix = [cos(pitch) 0 -sin(pitch);
                    0           1           0;
                    sin(pitch) 0  cos(pitch)];
    roll_matrix = [1            0           0;
                    0          cos(roll)    sin(roll);
                    0           -sin(roll)  cos(roll)];
    ZYXDCM = roll_matrix*pitch_matrix*yaw_matrix;
end

== matlab function ame532Project1_GimbalDynamicsModel/Gimbal Aircraft dynamic sim/translational dynamics/MATLAB Function10 ==
  data: p input; Cross_Product_Matrix output; q input; r input
function Cross_Product_Matrix = omega_to_cross_product_matrix(p,q,r)

    Cross_Product_Matrix =[0 -r q; r 0 -p; -q p 0];

end

== matlab function ame532Project1_GimbalDynamicsModel/Gimbal Aircraft dynamic sim/aeroforce coefficient block/MATLAB Function ==
  data: AR_matrix input; CL_a output
function CL_a = Calculate_CL_a(AR_matrix)

CL_a = zeros(4,1);

for i = 1:4
    CL_a(i) = 2*pi*(AR_matrix(i)/(2+AR_matrix(i)));
end

== matlab function ame532Project1_GimbalDynamicsModel/Gimbal Aircraft dynamic sim/Translational Kinematics/new C_EN base on cart. coordinate1 ==
  data: lat input; ZYXDCM output; long input
function ZYXDCM = DCM_from_Euler(lat,long) % sequence of rotation is lat long
%     yaw_matrix = [cos(yaw) sin(yaw) 0;
%                   -sin(yaw) cos(yaw) 0;
%                   0 0 1];
    lat_matrix = [cos(lat) 0 -sin(lat);
                    0           1           0;
                    sin(lat) 0  cos(lat)];
    long_matrix = [1            0           0;
                    0          cos(-long)    sin(-long);
                    0           -sin(-long)  cos(-long)];

    adjust_matrix = [cos(pi/2) 0 -sin(pi/2);
                    0           1           0;
                    sin(pi/2) 0  cos(pi/2)];
    ZYXDCM = adjust_matrix*long_matrix*lat_matrix;
end

%this rotational matrix turns lat long coordinate into a new C_EN
%assuming the N CS is lat and longitudinally rotated, then you would do
%-longditudinal rotation then lat rotation, then rotate 90 degrees again to
%match ECEF

== matlab function ame532Project1_GimbalDynamicsModel/Gimbal Aircraft dynamic sim/measurement subsystem/MATLAB Function ==
  data: velocity input; magnitude output
function magnitude = magnitude_from_vector(velocity)

magnitude = sqrt(velocity(1)^2+velocity(2)^2+velocity(3)^2);

end

== matlab function ame532Project1_GimbalDynamicsModel/Gimbal Aircraft dynamic sim/Translational Kinematics/C_EN from LAX to ECEF ==
  data: lat input; ZYXDCM output; long input
function ZYXDCM = DCM_from_Euler(lat,long) % sequence of rotation is lat long
%     yaw_matrix = [cos(yaw) sin(yaw) 0;
%                   -sin(yaw) cos(yaw) 0;
%                   0 0 1];
    lat_matrix = [cos(lat) 0 -sin(lat);
                    0           1           0;
                    sin(lat) 0  cos(lat)];
    long_matrix = [1            0           0;
                    0          cos(-long)    sin(-long);
                    0           -sin(-long)  cos(-long)];

    adjust_matrix = [cos(pi/2) 0 -sin(pi/2);
                    0           1           0;
                    sin(pi/2) 0  cos(pi/2)];
    ZYXDCM = adjust_matrix*long_matrix*lat_matrix;
end

%this rotational matrix turns lat long coordinate into a new C_EN
%assuming the N CS is lat and longitudinally rotated, then you would do
%-longditudinal rotation then lat rotation, then rotate 90 degrees again to
%match ECEF

== matlab function ame532Project1_GimbalDynamicsModel/Gimbal Aircraft dynamic sim/mass & aero property calculation/CG calculation ==
  data: M_matrix input; cg_x output; cg_y output; cg_z output
function [cg_x, cg_y, cg_z] = CG_calc(M_matrix)

mass_col = M_matrix(:,1);
x_col = M_matrix(:,5);
y_col = M_matrix(:,6);
z_col = M_matrix(:,7);

cg_x = sum(mass_col.*x_col)/(sum(mass_col));
cg_y = sum(mass_col.*y_col)/(sum(mass_col));
cg_z = sum(mass_col.*z_col)/(sum(mass_col));

end

== matlab function ame532Project1_GimbalDynamicsModel/Gimbal Aircraft dynamic sim/mass & aero property calculation/MATLAB Function ==
  data: cg_location input; M_matrix input; J_matrix output
function J_matrix = fcn(cg_location,M_matrix)


mass_col = M_matrix(:,1);
x_dim = M_matrix(:,2);
y_dim = M_matrix(:,3);
z_dim = M_matrix(:,4);
x_loc = M_matrix(:,5);
y_loc = M_matrix(:,6);
z_loc = M_matrix(:,7);

Ixx = zeros(11,1);
Iyy = zeros(11,1);
Izz = zeros(11,1);
Ixz = zeros(11,1);
Izx = Ixz;
Ixy = zeros(11,1);
Iyx = Ixy;
Iyz = zeros(11,1);
Izy = Iyz;

J_matrix = zeros(3,3);

% all moment of inertial is calculated wrt to CG

for i = 1:11
    Ixx(i) = mass_col(i)*(y_dim(i)^2+z_dim(i)^2)/(12)+mass_col(i)*((y_loc(i)-cg_location(2))^2+(z_loc(i)-cg_location(3))^2); % check discussion post
    Iyy(i) = mass_col(i)*(x_dim(i)^2+z_dim(i)^2)/(12)+mass_col(i)*((x_loc(i)-cg_location(1))^2+(z_loc(i)-cg_location(3))^2);
    Izz(i) = mass_col(i)*(y_dim(i)^2+x_dim(i)^2)/(12)+mass_col(i)*((y_loc(i)-cg_location(2))^2+(x_loc(i)-cg_location(1))^2);
    Ixz(i) = mass_col(i)*((z_loc(i)-cg_location(3))*(x_loc(i)-cg_location(1)));
    Ixy(i) = mass_col(i)*((x_loc(i)-cg_location(1))*(y_loc(i)-cg_location(2)));
    Iyz(i) = mass_col(i)*((y_loc(i)-cg_location(2))*(z_loc(i)-cg_location(3)));


end

J_matrix(1,1) = sum(Ixx);
J_matrix(2,2) = sum(Iyy);
J_matrix(3,3) = sum(Izz);
J_matrix(1,2) = sum(Ixy);
J_matrix(2,1) = sum(Ixy);
J_matrix(1,3) = sum(Ixz);
J_matrix(3,1) = sum(Ixz);
J_matrix(2,3) = sum(Iyz);
J_matrix(3,2) = sum(Iyz);

J_matrix = J_matrix./1000;
end

== matlab function ame532Project1_GimbalDynamicsModel/Gimbal Aircraft dynamic sim/mass & aero property calculation/MATLAB Function2 ==
  data: M_matrix input; aero_prop output
function aero_prop = fcn(M_matrix)

aero_prop = zeros(4,7);
for i = 1:4
    aero_prop(i,1:3) = M_matrix(i,5:7);
    aero_prop(i,4) = M_matrix(i,2);
end

%% define span for each surface

    aero_prop(1,5) = M_matrix(1,3); %right wing
    aero_prop(2,5) = M_matrix(2,3); %left wing
    aero_prop(3,5) = M_matrix(3,3); %hor stab.
    aero_prop(4,5) = M_matrix(4,4); %ver stab.
%% define area and aspect ratio for each surface

for i = 1:4
    aero_prop(i,6) = aero_prop(i,4)*aero_prop(i,5);
    aero_prop(i,7) = aero_prop(i,5)/aero_prop(i,4);
end

== matlab function ame532Project1_GimbalDynamicsModel/Gimbal Aircraft dynamic sim/aeroforce coefficient block/extract matrix function ==
  data: aero_surface_matrix input; AR_matrix output
function AR_matrix = Extract_AR(aero_surface_matrix)

AR_matrix = aero_surface_matrix(:,7);
end

== matlab function ame532Project1_GimbalDynamicsModel/Gimbal Aircraft dynamic sim/aeroforce coefficient block/calculatie alpha ==
  data: i0 input; alpha output; v_B input; n_vector input; wind_w input; v_B_BA output; C_BN input
function [alpha,v_B_BA] = fcn(i0,v_B,n_vector,wind_w,C_BN)

alpha = zeros(4,1);
% this function calculates alpha that the aero surface sees

v_B_BA = v_B - C_BN*wind_w;

for i = 1:4
    alpha(i) = i0(i) - asin(dot(v_B_BA,n_vector(:,i))/norm(v_B_BA));
end

== matlab function ame532Project1_GimbalDynamicsModel/Gimbal Aircraft dynamic sim/aeroforce coefficient block/MATLAB Function1 ==
  data: CL0 input; CL_s output; CL_a input; alpha input
function CL_s = calculate_CL_s(CL0,CL_a,alpha)

CL_s = zeros(4,1);

for i = 1:4
    CL_s(i) = CL0(i)+CL_a(i)*alpha(i);
end

== matlab function ame532Project1_GimbalDynamicsModel/Gimbal Aircraft dynamic sim/aeroforce coefficient block/MATLAB Function2 ==
  data: CD_0 input; CD_a input; CD_s output; alpha_0 input; alpha input; CL_s input; e input; AR input
function CD_s = calculate_CD_s(CD_0,CD_a,alpha_0,alpha,CL_s,e,AR)
CD_s = zeros(4,1);

for i = 1:4
    
    CD_s(i) = CD_0(i) + CD_a(i)*(alpha(i)-alpha_0(i))^2+(CL_s(i)^2)/(pi*e(i)*AR(i));

end

== matlab function ame532Project1_GimbalDynamicsModel/Gimbal Aircraft dynamic sim/aeroforce coefficient block/extract matrix function1 ==
  data: aero_surface_matrix input; AR_matrix output
function AR_matrix = Extract_AR(aero_surface_matrix)

AR_matrix = aero_surface_matrix(:,7);
end

== matlab function ame532Project1_GimbalDynamicsModel/Gimbal Aircraft dynamic sim/aeroforce coefficient block/MATLAB Function3 ==
  data: alpha input; CM_0 input; CM_s output; CM_a input
function CM_s = calculate_CM_s(alpha,CM_0,CM_a)

CM_s = zeros(4,1);

for i = 1:4
    CM_s(i) = CM_0(i)+CM_a(i)*alpha(i);
end

== matlab function ame532Project1_GimbalDynamicsModel/IMU  Aircraft dynamic sim1/Rotational Kinematics/C_BN ==
  data: roll input; ZYXDCM output; pitch input; yaw input
function ZYXDCM = DCM_from_Euler(roll,pitch,yaw) % sequence is yaw pitch roll
    yaw_matrix = [cos(yaw) sin(yaw) 0;
                  -sin(yaw) cos(yaw) 0;
                  0 0 1];
    pitch_matrix = [cos(pitch) 0 -sin(pitch);
                    0           1           0;
                    sin(pitch) 0  cos(pitch)];
    roll_matrix = [1            0           0;
                    0          cos(roll)    sin(roll);
                    0           -sin(roll)  cos(roll)];
    ZYXDCM = roll_matrix*pitch_matrix*yaw_matrix;
end

== matlab function ame532Project1_GimbalDynamicsModel/Gimbal Aircraft dynamic sim/aeroforce & moment block/MATLAB Function ==
  data: CL_s input; Lift_s output; totalspeed input; area_s input
function Lift_s = calculate_Lift_s(CL_s,totalspeed,area_s)

Lift_s = zeros(4,1);
rho = 1.225; %kg/m3

for i = 1:4
    Lift_s(i) = CL_s(i)*0.5*rho*(totalspeed^2)*area_s(i);
end

end

== matlab function ame532Project1_GimbalDynamicsModel/Gimbal Aircraft dynamic sim/aeroforce & moment block/MATLAB Function1 ==
  data: aerosurface_matrix input; area_col output
function area_col = extract_area_col(aerosurface_matrix)

area_col = aerosurface_matrix(:,6);

end

== matlab function ame532Project1_GimbalDynamicsModel/Gimbal Aircraft dynamic sim/aeroforce & moment block/MATLAB Function2 ==
  data: CD_s input; Drag_s output; totalspeed input; area_s input
function Drag_s = calculate_Drag_s(CD_s,totalspeed,area_s)

Drag_s = zeros(4,1);
rho = 1.225; %kg/m3

for i = 1:4
    Drag_s(i) = CD_s(i)*0.5*rho*(totalspeed^2)*area_s(i);
end

end

== matlab function ame532Project1_GimbalDynamicsModel/Gimbal Aircraft dynamic sim/aeroforce & moment block/MATLAB Function3 ==
  data: CM_s input; Moment_s output; totalspeed input; area_s input; chord_s input
function Moment_s = calculate_Moment_s(CM_s,totalspeed,area_s,chord_s)

Moment_s = zeros(4,1);
rho = 1.225; %kg/m3

for i = 1:4
    Moment_s(i) = CM_s(i)*0.5*rho*(totalspeed^2)*area_s(i)*chord_s(i);
end

end

== matlab function ame532Project1_GimbalDynamicsModel/Gimbal Aircraft dynamic sim/aeroforce & moment block/MATLAB Function4 ==
  data: aerosurface_matrix input; chord_col output
function chord_col = extract_chord_col(aerosurface_matrix)

chord_col = aerosurface_matrix(:,4);

end

== matlab function ame532Project1_GimbalDynamicsModel/Gimbal Aircraft dynamic sim/aeroforce & moment block/MATLAB Function5 ==
  data: Lift_s input; F_w_s output; n_vector_s input; Drag_s input
function F_w_s = Calculate_F_w(Lift_s,n_vector_s,Drag_s)

F_w_s = zeros(3,4);

for i = 1:4
    F_w_s(:,i) = Lift_s(i).*n_vector_s(:,i) - [Drag_s(i) 0 0]';
end

== matlab function ame532Project1_GimbalDynamicsModel/Gimbal Aircraft dynamic sim/aeroforce & moment block/MATLAB Function6 ==
  data: n_vector_s input; M_s input; M_w_s output; F_b_s input; x_b_sb input
function M_w_s = Calculate_M_w(n_vector_s,M_s,F_b_s,x_b_sb)

M_w_s = zeros(3,4);

for i = 1:4
      M_w_s(:,i) = M_s(i)*[0 0 0; 0 0 -1; 0 1 0]*n_vector_s(:,i)+cross(x_b_sb(:,i),F_b_s(:,i));
%     M_w_s(:,i) = M_s(i)*[0 0 0; 0 0 -1; 0 1 0]*n_vector_s(:,i)+cross(F_b_s(:,i),x_b_sb(:,i));

end

== matlab function ame532Project1_GimbalDynamicsModel/Gimbal Aircraft dynamic sim/mass & aero property calculation/MATLAB Function1 ==
  data: aero_prop_matrix input; m_matrix input; x_b_s_ac output; cg_location input
function x_b_s_ac = calculate_x_b_sb(aero_prop_matrix,m_matrix,cg_location)
%this function calculates vector of each component to CM of aircraft

x_b_sb = zeros(3,4);
x_b_s_ac = zeros(3,4);
for i = 1:4
    x_b_s_ac(:,i) = m_matrix(i,5:7)' + [0.25*aero_prop_matrix(i,4) 0 0]';
    x_b_s_ac(:,i) = x_b_s_ac(:,i)- cg_location;

%     x_b_sb(:,i) = m_matrix(i,5:7)' - cg_location;

end

== matlab function ame532Project1_GimbalDynamicsModel/Gimbal Aircraft dynamic sim/aeroforce & moment block/MATLAB Function7 ==
  data: forcexyz_w_s_matrix input; force_xyz_w output
function force_xyz_w = sum_all_force_xyz(forcexyz_w_s_matrix)

force_xyz_w = zeros(3,1);

for i = 1:3
    force_xyz_w(i) = sum(forcexyz_w_s_matrix(i,:));
end

== matlab function ame532Project1_GimbalDynamicsModel/Gimbal Aircraft dynamic sim/aeroforce & moment block/MATLAB Function8 ==
  data: m_b_s input; moments_lmn_b output
function moments_lmn_b = sum_all_moments_b_s(m_b_s)

moments_lmn_b = zeros(3,1);

for i = 1:3
    moments_lmn_b(i) = sum(m_b_s(i,:));
end

== matlab function ame532Project1_GimbalDynamicsModel/Gimbal Aircraft dynamic sim/aeroforce & moment block/MATLAB Function9 ==
  data: DCM_WB output; v_body_ba input; alpha output; beta output; v_inf output
function [DCM_WB,alpha,beta,v_inf]  = construct_DCM_bw(v_body_ba)

alpha = atan2(v_body_ba(3),v_body_ba(1));
beta = asin(v_body_ba(2)/norm(v_body_ba));

DCM_WB = [cos(beta) sin(beta) 0; -sin(beta) cos(beta) 0; 0 0 1]*[cos(alpha) 0 sin(alpha); 0 1 0; -sin(alpha) 0 cos(alpha)];
v_inf = norm(v_body_ba);
end

== matlab function ame532Project1_GimbalDynamicsModel/IMU  Aircraft dynamic sim1/Rotational Kinematics/C_EN1 ==
  data: roll input; ZYXDCM output; pitch input; yaw input
function ZYXDCM = DCM_from_Euler(roll,pitch,yaw) % sequence is yaw pitch roll
    yaw_matrix = [cos(yaw) sin(yaw) 0;
                  -sin(yaw) cos(yaw) 0;
                  0 0 1];
    pitch_matrix = [cos(pitch) 0 -sin(pitch);
                    0           1           0;
                    sin(pitch) 0  cos(pitch)];
    roll_matrix = [1            0           0;
                    0          cos(roll)    sin(roll);
                    0           -sin(roll)  cos(roll)];
    ZYXDCM = roll_matrix*pitch_matrix*yaw_matrix;
end

== matlab function ame532Project1_GimbalDynamicsModel/IMU  Aircraft dynamic sim1/Rotational Kinematics/MATLAB Function3 ==
  data: p input; Cross_Product_Matrix output; q input; r input
function Cross_Product_Matrix = omega_to_cross_product_matrix(p,q,r)

    Cross_Product_Matrix =[0 -r q; r 0 -p; -q p 0];

end

== matlab function ame532Project1_GimbalDynamicsModel/IMU  Aircraft dynamic sim1/Rotational Kinematics/MATLAB Function4 ==
  data: DCM input; roll output; pitch output; yaw output
function [roll, pitch, yaw] = Euler_from_DCM(DCM)
   roll = atan2(DCM(2,3),DCM(3,3));
   pitch = -asin(DCM(1,3));
   yaw = atan2(DCM(1,2),DCM(1,1));
end

== matlab function ame532Project1_GimbalDynamicsModel/IMU  Aircraft dynamic sim1/Rotational Kinematics/MATLAB Function5 ==
  data: DCM input; roll output; pitch output; yaw output
function [roll, pitch, yaw] = Euler_from_DCM(DCM)
   roll = atan2(DCM(2,3),DCM(3,3));
   pitch = asin(DCM(1,3));
   yaw = atan2(DCM(1,2),DCM(1,1));
end

== matlab function ame532Project1_GimbalDynamicsModel/IMU  Aircraft dynamic sim1/Rotational Kinematics/MATLAB Function6 ==
  data: DCM input; roll output; pitch output; yaw output
function [roll, pitch, yaw] = Euler_from_DCM(DCM)
   roll = atan2(DCM(2,3),DCM(3,3));
   pitch = -asin(DCM(1,3));
   yaw = atan2(DCM(1,2),DCM(1,1));
end

== matlab function ame532Project1_GimbalDynamicsModel/IMU  Aircraft dynamic sim1/Rotational Kinematics/MATLAB Function7 ==
  data: quat input; roll output; pitch output; yaw output
function [roll, pitch, yaw] = Euler_from_Quat(quat)
    DCM = zeros(3,3);
    DCM(1) = (quat(1)^2+quat(2)^2-quat(3)^2-quat(4)^2);
    DCM(2) = 2*(quat(2)*quat(3)-quat(1)*quat(4));
    DCM(3) = 2*(quat(2)*quat(4)+quat(1)*quat(3));
    DCM(4) = 2*(quat(2)*quat(3)+quat(1)*quat(4));
    DCM(5) = (quat(1)^2-quat(2)^2+quat(3)^2-quat(4)^2);
    DCM(6) = 2*(quat(3)*quat(4)-quat(1)*quat(2));
    DCM(7) = 2*(quat(2)*quat(4)-quat(1)*quat(3));
    DCM(8) = 2*(quat(3)*quat(4)+quat(1)*quat(2));
    DCM(9) = (quat(1)^2-quat(2)^2-quat(3)^2+quat(4)^2);

    roll = atan2(DCM(2,3),DCM(3,3));
    pitch = -asin(DCM(1,3));
    yaw = atan2(DCM(1,2),DCM(1,1));
end

== matlab function ame532Project1_GimbalDynamicsModel/IMU  Aircraft dynamic sim1/Rotational Kinematics/MATLAB Function8 ==
  data: roll input; ZYXquat_inv output; pitch input; yaw input; ZYXquat output
function [ZYXquat_inv,ZYXquat] = Quat_from_Euler(roll,pitch,yaw)
    q_yaw = zeros(4,1);
    q_yaw(1) = cos(yaw/2);
    q_yaw(2:4,1) = sin(yaw/2)*[0 0 1]';

    q_pitch = zeros(4,1);
    q_pitch(1) = cos(pitch/2);
    q_pitch(2:4,1) = sin(pitch/2)*[0 1 0]';

    q_roll = zeros(4,1);
    q_roll(1) = cos(roll/2);
    q_roll(2:4,1) = sin(roll/2)*[1 0 0]';
    
    inv_q_yaw = [q_yaw(1);-q_yaw(2:4)];
    inv_q_pitch = [q_pitch(1);-q_pitch(2:4)];
    inv_q_roll = [q_roll(1);-q_roll(2:4)];

    ZYXquat_inv = quat_mult(quat_mult(inv_q_roll,inv_q_pitch),inv_q_yaw);
    ZYXquat = quat_mult(quat_mult(q_yaw,q_pitch),q_roll);

end

function quat = quat_mult(q1,q2)
    quat = zeros(4,1);
    quat(1) = q1(1)*q2(1)-q1(2)*q2(2)-q1(3)*q2(3)-q1(4)*q2(4);
    quat(2) = q1(1)*q2(2)+q1(2)*q2(1)+q1(3)*q2(4)-q1(4)*q2(3);
    quat(3) = q1(1)*q2(3)-q1(2)*q2(4)+q1(3)*q2(1)+q1(4)*q2(2);
    quat(4) = q1(1)*q2(4)+q1(2)*q2(3)-q1(3)*q2(2)+q1(4)*q2(1);
end

== matlab function ame532Project1_GimbalDynamicsModel/IMU  Aircraft dynamic sim1/Rotational Kinematics/MATLAB Function9 ==
  data: q1 input; quat output; q2 input
function quat = quat_mult(q1,q2)
    quat = zeros(4,1);
    quat(1) = q1(1)*q2(1)-q1(2)*q2(2)-q1(3)*q2(3)-q1(4)*q2(4);
    quat(2) = q1(1)*q2(2)+q1(2)*q2(1)+q1(3)*q2(4)-q1(4)*q2(3);
    quat(3) = q1(1)*q2(3)-q1(2)*q2(4)+q1(3)*q2(1)+q1(4)*q2(2);
    quat(4) = q1(1)*q2(4)+q1(2)*q2(3)-q1(3)*q2(2)+q1(4)*q2(1);
end

== matlab function ame532Project1_GimbalDynamicsModel/IMU  Aircraft dynamic sim1/Translational Kinematics/C_EN from LAX to ECEF ==
  data: lat input; ZYXDCM output; long input
function ZYXDCM = DCM_from_Euler(lat,long) % sequence of rotation is lat long
%     yaw_matrix = [cos(yaw) sin(yaw) 0;
%                   -sin(yaw) cos(yaw) 0;
%                   0 0 1];
    lat_matrix = [cos(lat) 0 -sin(lat);
                    0           1           0;
                    sin(lat) 0  cos(lat)];
    long_matrix = [1            0           0;
                    0          cos(-long)    sin(-long);
                    0           -sin(-long)  cos(-long)];

    adjust_matrix = [cos(pi/2) 0 -sin(pi/2);
                    0           1           0;
                    sin(pi/2) 0  cos(pi/2)];
    ZYXDCM = adjust_matrix*long_matrix*lat_matrix;
end

%this rotational matrix turns lat long coordinate into a new C_EN
%assuming the N CS is lat and longitudinally rotated, then you would do
%-longditudinal rotation then lat rotation, then rotate 90 degrees again to
%match ECEF
